simulink model "SafaeeModel"  (R2021a)
settings: Solver=VariableStepAuto  StartTime=0.0  StopTime=10  RelTol=1e-3
libraries: fuzblock x6
settings Model: Creator=carlos  LastModifiedBy=Lenovo
settings SolverCC: AlgebraicLoopSolver=TrustRegion
settings DataIOCC: ReturnWorkspaceOutputs=off
settings DebuggingCC: SFMachineParentedDataDiag=warning  ArithmeticOperatorsInVariantConditions=warning
settings SFSimCC: CustomCodeUndefinedFunction=UseInterfaceOnly

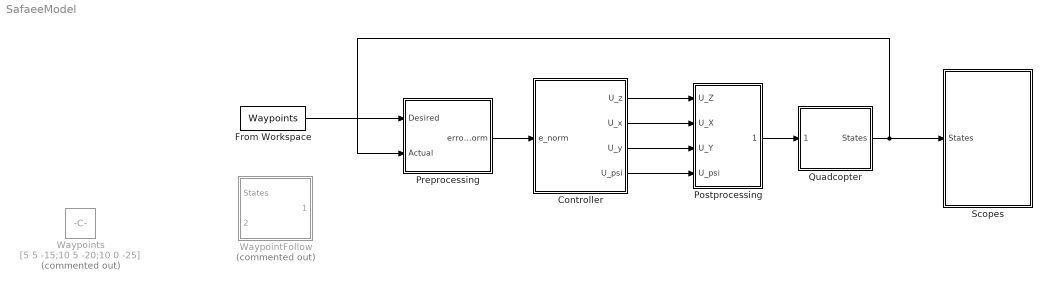
== system SafaeeModel ==
  Controller : Subsystem
  From Workspace : FromWorkspace  VariableName=Waypoints
  Postprocessing : Subsystem
  Preprocessing : Subsystem
  Quadcopter : Subsystem
  Scopes : Subsystem
  WaypointFollow : Subsystem  Commented=on
  Waypoints : Constant  Commented=on  Value=[5 5 -15;10 5 -20;10 0 -25]  VectorParams1D=off
  wires:
  Preprocessing/1(errorNorm) -> Controller/1(e_norm)
  Controller/1(U_z) -> Postprocessing/1(U_Z)
  Controller/2(U_x) -> Postprocessing/2(U_X)
  Controller/3(U_y) -> Postprocessing/3(U_Y)
  Controller/4(U_psi) -> Postprocessing/4(U_psi)
  Postprocessing/1(Omegas) -> Quadcopter/1(Omegas)
  Quadcopter/1(States) -> Preprocessing/2(Actual), Scopes/1(States)
  From Workspace/1 -> Preprocessing/1(Desired)

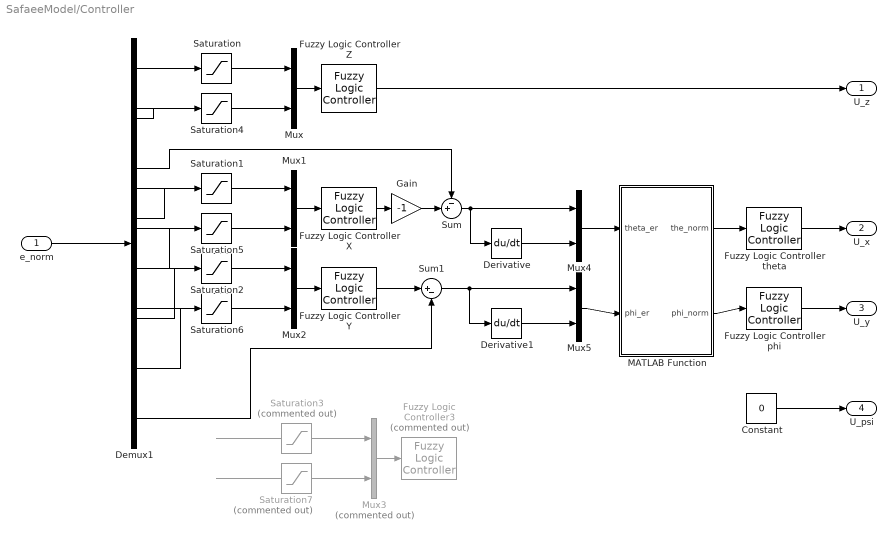
== system SafaeeModel/Controller ==
  e_norm : Inport
  Constant : Constant  Value=0
  Demux1 : Demux  Outputs=8
  Derivative : Derivative  CoefficientInTFapproximation=1
  Derivative1 : Derivative  CoefficientInTFapproximation=1
  Fuzzy Logic Controller X : fuzblock/Fuzzy Logic  Controller  FIS=FLCs.FLC_X  OutputSampleNumber=101  DataType=double  FuzzifiedInputs=off  RuleFiringStrengths=off  RuleOutputs=off  AggregatedOutputs=off  SimulateUsing=Interpreted execution  OutOfRangeInputValueMessage=warning  NoRuleFiredMessage=warning  EmptyOutputFuzzySetMessage=warning
  Fuzzy Logic Controller Y : fuzblock/Fuzzy Logic  Controller  FIS=FLCs.FLC_Y  OutputSampleNumber=101  DataType=double  FuzzifiedInputs=off  RuleFiringStrengths=off  RuleOutputs=off  AggregatedOutputs=off  SimulateUsing=Interpreted execution  OutOfRangeInputValueMessage=warning  NoRuleFiredMessage=warning  EmptyOutputFuzzySetMessage=warning
  Fuzzy Logic Controller Z : fuzblock/Fuzzy Logic  Controller  FIS=FLCs.FLC_Z  OutputSampleNumber=101  DataType=double  FuzzifiedInputs=off  RuleFiringStrengths=off  RuleOutputs=off  AggregatedOutputs=off  SimulateUsing=Interpreted execution  OutOfRangeInputValueMessage=warning  NoRuleFiredMessage=warning  EmptyOutputFuzzySetMessage=warning
  Fuzzy Logic Controller phi : fuzblock/Fuzzy Logic  Controller  FIS=FLCs.FLC_phi  OutputSampleNumber=101  DataType=double  FuzzifiedInputs=off  RuleFiringStrengths=off  RuleOutputs=off  AggregatedOutputs=off  SimulateUsing=Interpreted execution  OutOfRangeInputValueMessage=warning  NoRuleFiredMessage=warning  EmptyOutputFuzzySetMessage=warning
  Fuzzy Logic Controller theta : fuzblock/Fuzzy Logic  Controller  FIS=FLCs.FLC_th  OutputSampleNumber=101  DataType=double  FuzzifiedInputs=off  RuleFiringStrengths=off  RuleOutputs=off  AggregatedOutputs=off  SimulateUsing=Interpreted execution  OutOfRangeInputValueMessage=warning  NoRuleFiredMessage=warning  EmptyOutputFuzzySetMessage=warning
  Fuzzy Logic Controller3 : fuzblock/Fuzzy Logic  Controller  Commented=on  FIS=FLCs.FLC_psi  OutputSampleNumber=101  DataType=double  FuzzifiedInputs=off  RuleFiringStrengths=off  RuleOutputs=off  AggregatedOutputs=off  SimulateUsing=Interpreted execution  OutOfRangeInputValueMessage=warning  NoRuleFiredMessage=warning  EmptyOutputFuzzySetMessage=warning
  Gain : Gain  Gain=-1
  MATLAB Function : MATLAB Function  TreatAsAtomicUnit=on
  Mux{,1..2,4..5} (5 alike) : Mux  Inputs=2
  Mux3 : Mux  Commented=on  Inputs=2
  Saturation : Saturate  UpperLimit=1  LowerLimit=-1  ZeroCross=off
  Saturation1 : Saturate  UpperLimit=1  LowerLimit=-1  ZeroCross=off
  Saturation2 : Saturate  UpperLimit=1  LowerLimit=-1  ZeroCross=off
  Saturation3 : Saturate  Commented=on  UpperLimit=1  LowerLimit=-1  ZeroCross=off
  Saturation4 : Saturate  UpperLimit=3  LowerLimit=-3  ZeroCross=off
  Saturation5 : Saturate  UpperLimit=3  LowerLimit=-3  ZeroCross=off
  Saturation6 : Saturate  UpperLimit=3  LowerLimit=-3  ZeroCross=off
  Saturation7 : Saturate  Commented=on  UpperLimit=3  LowerLimit=-3  ZeroCross=off
  Sum : Sum  Inputs=-+|
  Sum1 : Sum  Inputs=|+-
  U_z : Outport  VectorParamsAs1DForOutWhenUnconnected=off
  U_x : Outport  Port=2  VectorParamsAs1DForOutWhenUnconnected=off
  U_y : Outport  Port=3  VectorParamsAs1DForOutWhenUnconnected=off
  U_psi : Outport  Port=4  VectorParamsAs1DForOutWhenUnconnected=off
  wires:
  Fuzzy Logic Controller Z/1 -> U_z/1
  Demux1/3 -> Sum/1
  Demux1/4 -> Saturation1/1
  Demux1/5 -> Saturation5/1
  Demux1/2 -> Saturation4/1
  e_norm/1 -> Demux1/1
  Demux1/1 -> Saturation/1
  Demux1/6 -> Saturation2/1
  Demux1/8 -> Sum1/2
  Demux1/7 -> Saturation6/1
  Fuzzy Logic Controller X/1 -> Gain/1
  Sum/1 -> Mux4/1, Derivative/1
  Fuzzy Logic Controller theta/1 -> U_x/1
  Fuzzy Logic Controller Y/1 -> Sum1/1
  Sum1/1 -> Mux5/1, Derivative1/1
  Fuzzy Logic Controller phi/1 -> U_y/1
  Mux/1 -> Fuzzy Logic Controller Z/1
  Mux2/1 -> Fuzzy Logic Controller Y/1
  Mux1/1 -> Fuzzy Logic Controller X/1
  Mux3/1 -> Fuzzy Logic Controller3/1
  Derivative/1 -> Mux4/2
  Mux4/1 -> MATLAB Function/1(theta_er)
  Derivative1/1 -> Mux5/2
  Mux5/1 -> MATLAB Function/2(phi_er)
  MATLAB Function/1(the_norm) -> Fuzzy Logic Controller theta/1
  MATLAB Function/2(phi_norm) -> Fuzzy Logic Controller phi/1
  Gain/1 -> Sum/2
  Saturation/1 -> Mux/1
  Saturation1/1 -> Mux1/1
  Saturation2/1 -> Mux2/1
  Saturation3/1 -> Mux3/1
  Saturation4/1 -> Mux/2
  Saturation5/1 -> Mux1/2
  Saturation6/1 -> Mux2/2
  Saturation7/1 -> Mux3/2
  Constant/1 -> U_psi/1

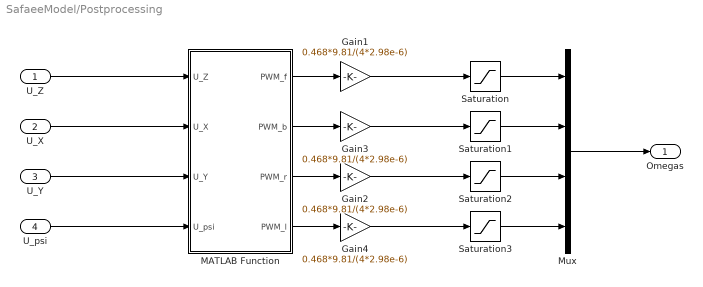
== system SafaeeModel/Postprocessing ==
  U_Z : Inport
  U_X : Inport  Port=2
  U_Y : Inport  Port=3
  U_psi : Inport  Port=4
  Gain{1..4} (4 alike) : Gain  Gain=0.468*9.81/(4*2.98e-6)
  MATLAB Function : MATLAB Function  TreatAsAtomicUnit=on
  Mux : Mux
  Saturation{,1..3} (4 alike) : Saturate  UpperLimit=1000000  LowerLimit=0  ZeroCross=off
  Omegas : Outport  VectorParamsAs1DForOutWhenUnconnected=off
  wires:
  Gain2/1 -> Saturation2/1
  Mux/1 -> Omegas/1
  Gain4/1 -> Saturation3/1
  MATLAB Function/4(PWM_l) -> Gain4/1
  MATLAB Function/2(PWM_b) -> Gain3/1
  Gain3/1 -> Saturation1/1
  MATLAB Function/3(PWM_r) -> Gain2/1
  Gain1/1 -> Saturation/1
  U_Y/1 -> MATLAB Function/3(U_Y)
  MATLAB Function/1(PWM_f) -> Gain1/1
  U_Z/1 -> MATLAB Function/1(U_Z)
  U_psi/1 -> MATLAB Function/4(U_psi)
  U_X/1 -> MATLAB Function/2(U_X)
  Saturation/1 -> Mux/1
  Saturation1/1 -> Mux/2
  Saturation2/1 -> Mux/3
  Saturation3/1 -> Mux/4

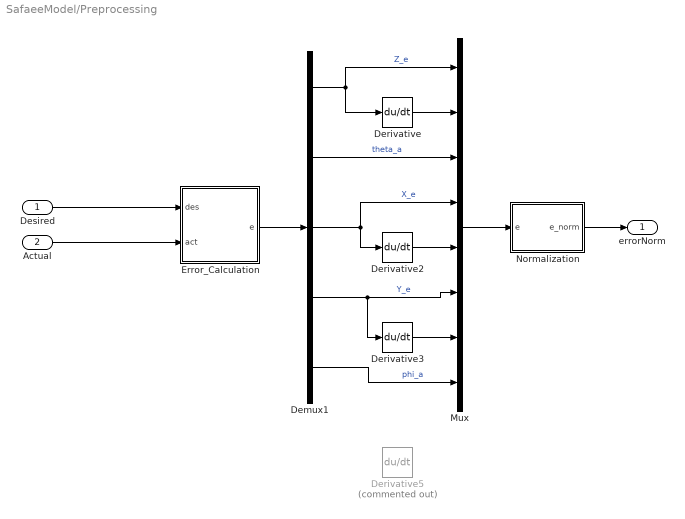
== system SafaeeModel/Preprocessing ==
  Desired : Inport
  Actual : Inport  Port=2
  Demux1 : Demux  Outputs=5
  Derivative : Derivative  CoefficientInTFapproximation=1
  Derivative2 : Derivative  CoefficientInTFapproximation=1
  Derivative3 : Derivative  CoefficientInTFapproximation=1
  Derivative5 : Derivative  Commented=on  CoefficientInTFapproximation=1
  Error_Calculation : MATLAB Function  TreatAsAtomicUnit=on
  Mux : Mux  Inputs=8
  Normalization : MATLAB Function  TreatAsAtomicUnit=on
  errorNorm : Outport  VectorParamsAs1DForOutWhenUnconnected=off
  wires:
  Demux1/1 -> Mux/1, Derivative/1  "Z_e"
  Demux1/2 -> Mux/3  "theta_a"
  Demux1/3 -> Mux/4, Derivative2/1  "X_e"
  Error_Calculation/1(e) -> Demux1/1
  Normalization/1(e_norm) -> errorNorm/1
  Demux1/4 -> Derivative3/1, Mux/6  "Y_e"
  Demux1/5 -> Mux/8  "phi_a"
  Mux/1 -> Normalization/1(e)
  Derivative2/1 -> Mux/5
  Derivative3/1 -> Mux/7
  Derivative/1 -> Mux/2
  Desired/1 -> Error_Calculation/1(des)
  Actual/1 -> Error_Calculation/2(act)

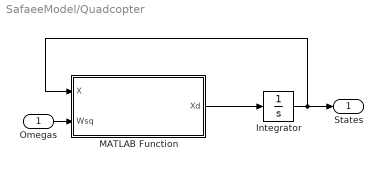
== system SafaeeModel/Quadcopter ==
  Omegas : Inport
  Integrator : Integrator  InitialCondition=[0;0;0;0;0;0;0;0;0;0;0;0]
  MATLAB Function : MATLAB Function  TreatAsAtomicUnit=on
  States : Outport  VectorParamsAs1DForOutWhenUnconnected=off
  wires:
  Omegas/1 -> MATLAB Function/2(Wsq)
  MATLAB Function/1(Xd) -> Integrator/1
  Integrator/1 -> States/1, MATLAB Function/1(X)

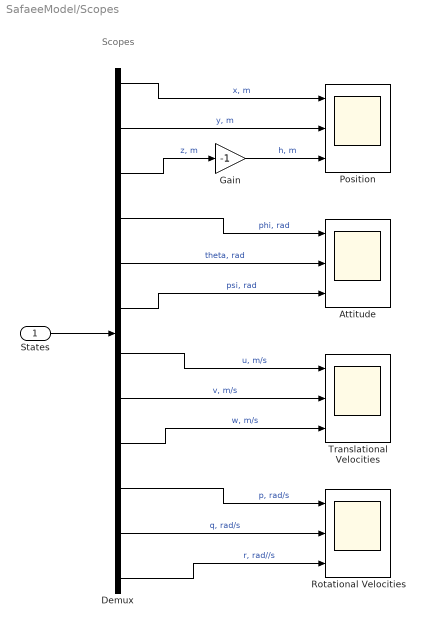
== system SafaeeModel/Scopes ==
  note: Scopes
  States : Inport
  Attitude : Scope  NumInputPorts=3
  Demux : Demux  Outputs=12
  Gain : Gain  Gain=-1
  Position : Scope  NumInputPorts=3
  Rotational Velocities : Scope  NumInputPorts=3
  Translational Velocities : Scope  NumInputPorts=3
  wires:
  Demux/5 -> Attitude/2  "theta, rad"
  Demux/1 -> Position/1  "x, m"
  Demux/4 -> Attitude/1  "phi, rad"
  Gain/1 -> Position/3  "h, m"
  Demux/6 -> Attitude/3  "psi, rad"
  Demux/11 -> Rotational Velocities/2  "q, rad/s"
  States/1 -> Demux/1
  Demux/3 -> Gain/1  "z, m"
  Demux/10 -> Rotational Velocities/1  "p, rad/s"
  Demux/12 -> Rotational Velocities/3  "r, rad//s"
  Demux/9 -> Translational Velocities/3  "w, m/s"
  Demux/8 -> Translational Velocities/2  "v, m/s"
  Demux/7 -> Translational Velocities/1  "u, m/s"
  Demux/2 -> Position/2  "y, m"

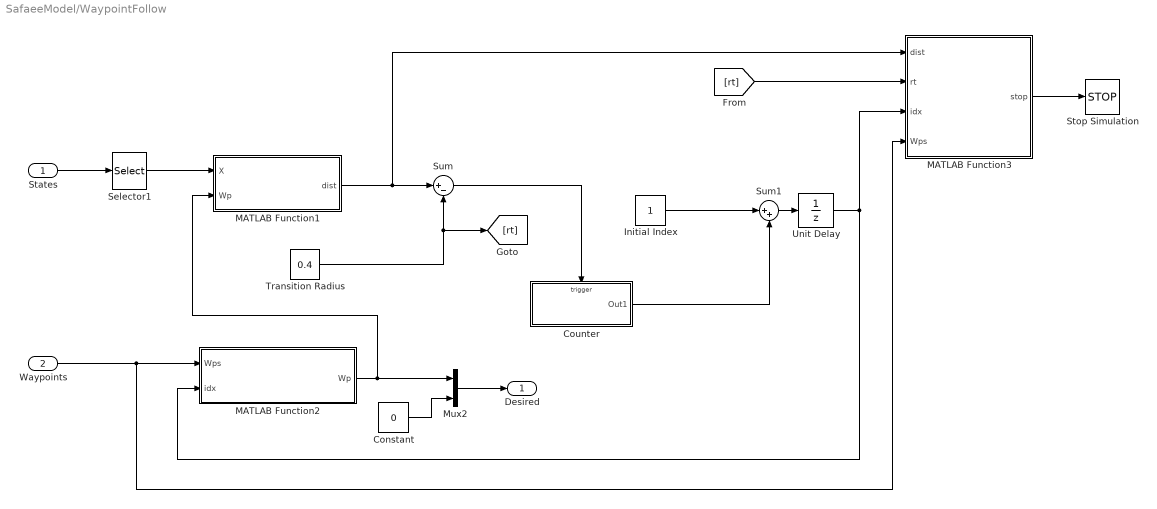
== system SafaeeModel/WaypointFollow ==
  States : Inport
  Waypoints : Inport  Port=2
  Constant : Constant  Value=0
  Counter : Subsystem  TreatAsAtomicUnit=on
  Initial Index : Constant
  MATLAB Function1 : MATLAB Function  TreatAsAtomicUnit=on
  MATLAB Function2 : MATLAB Function  TreatAsAtomicUnit=on
  MATLAB Function3 : MATLAB Function  TreatAsAtomicUnit=on
  Mux2 : Mux  Inputs=2
  Selector1 : Selector  InputPortWidth=12  IndexOptions=Index vector (dialog)  Indices=[1 2 3]  OutputSizes=1
  Stop Simulation : Stop
  Sum : Sum  Inputs=|+-
  Sum1 : Sum  Inputs=|++
  Transition Radius : Constant  Value=0.4
  Unit Delay : UnitDelay  InitialCondition=1  SampleTime=-1  HasFrameUpgradeWarning=on
  Desired : Outport
  wires:
  States/1 -> Selector1/1
  Selector1/1 -> MATLAB Function1/1(X)
  Transition Radius/1 -> [rt], Sum/2
  Sum/1 -> Counter/Trigger
  Counter/1(Out1) -> Sum1/2
  Initial Index/1 -> Sum1/1
  MATLAB Function2/1(Wp) -> Mux2/1, MATLAB Function1/2(Wp)
  Sum1/1 -> Unit Delay/1
  [rt] -> MATLAB Function3/2(rt)
  Waypoints/1 -> MATLAB Function2/1(Wps), MATLAB Function3/4(Wps)
  MATLAB Function3/1(stop) -> Stop Simulation/1
  Mux2/1 -> Desired/1
  Constant/1 -> Mux2/2
  Unit Delay/1 -> MATLAB Function2/2(idx), MATLAB Function3/3(idx)
  MATLAB Function1/1(dist) -> MATLAB Function3/1(dist), Sum/1

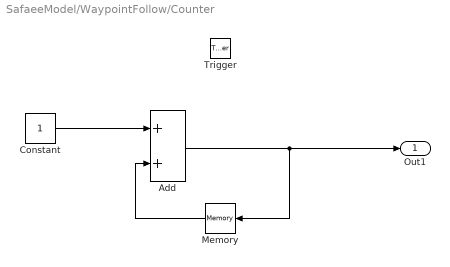
== system SafaeeModel/WaypointFollow/Counter ==
  Trigger : TriggerPort  TriggerType=falling  VariantControl=(inherit)
  Add : Sum
  Constant : Constant
  Memory : Memory  InheritSampleTime=on
  Out1 : Outport
  wires:
  Constant/1 -> Add/1
  Add/1 -> Memory/1, Out1/1
  Memory/1 -> Add/2

== matlab function SafaeeModel/Preprocessing/Error_Calculation ==
  data: des input; e output; act input
function e = fcn(des, act)

X_des = des(1,1); Y_des = des(1,2); Z_des = des(1,3);
% phi_des = des(4,1); theta_des = des(5,1); 
% psi_des = des(4,1);

X_act = act(1,1); Y_act = act(2,1); Z_act = act(3,1);
phi_act = act(4,1); theta_act = act(5,1); 
% psi_act = act(6,1);

ex      = X_des - X_act;
ey      = Y_des - Y_act;
ez      = Z_des - Z_act;
% ephi    = phi_des - phi_act;
% etheta  = theta_des - theta_act;
% epsi    = psi_des - psi_act;

e = [ez; theta_act; ex; ey; phi_act];% epsi];

== matlab function SafaeeModel/Quadcopter/MATLAB Function ==
  data: X input; Xd output; Wsq input
function Xd = Quadcopter(X, Wsq)
% Parameters from Luukkonen
g = 9.81;
M = 0.468;
Jx = 4.856e-3;
Jy = 4.856e-3;
Jz = 8.801e-3;
l = 0.225;
KT = 2.980e-6;
Kt = 1.140e-7;

% States
x   = X(1,1);  y   = X(2,1);  z   = X(3,1);
phi = X(4,1);  the = X(5,1);  psi = X(6,1);
u   = X(7,1);  v   = X(8,1);  w   = X(9,1);
p   = X(10,1); q   = X(11,1); r   = X(12,1);

% Motor Forces (front, back, right, left)
Tf   = KT*Wsq(1,1);  Tb   = KT*Wsq(2,1);   Tr   = KT*Wsq(3,1);  Tl   = KT*Wsq(4,1);

% Motor Torques (front, back, right, left)
tauf = -Kt*Wsq(1,1);  taub = -Kt*Wsq(2,1);  taur = Kt*Wsq(3,1);  taul = Kt*Wsq(4,1);

%% Safaee's quadcopter model
% Elements of Rotation Matrix from Inertial frame to Body Frame (Transposed)
R11 = cos(phi)*cos(psi);
R12 = sin(phi)*sin(the)*cos(psi) - cos(phi)*sin(psi);
R13 = cos(phi)*sin(the)*cos(psi) + sin(phi)*sin(psi);
R21 = cos(the)*sin(psi);
R22 = sin(phi)*sin(the)*sin(psi) + cos(phi)*cos(psi);
R23 = cos(phi)*sin(the)*sin(psi) - sin(phi)*cos(psi);
R31 = -sin(the);
R32 = sin(phi)*cos(the);
R33 = cos(phi)*cos(the);

% Rotation Matrix from Inertial frame to Body Frame (Transposed)
RI2BT = [R11 R12 R13;
         R21 R22 R23;
         R31 R32 R33];

% Translational Kinematics
Xd1 = RI2BT*[u; v; w];

% Elements of Rotational Kinematics Matrix
RE1 = 1;
RE2 = sin(phi)*tan(the);
RE3 = cos(phi)*tan(the);
RE4 = 0;
RE5 = cos(phi);
RE6 = -sin(phi);
RE7 = 0;
RE8 = sin(phi)./cos(the);
RE9 = cos(phi)./cos(the);

% Rotational Kinematics Matrix
RE = [RE1 RE2 RE3;
      RE4 RE5 RE6;
      RE7 RE8 RE9];
  
% Rotational Kinematics
Xd2 = RE*[p; q; r];

% Total Thrust
Tt = Tf + Tb + Tr + Tl;

% Total Torque along x axis
Tphi = l*(Tl - Tr);

% Total Torque along y axis
Tthe = l*(Tf - Tb);

% Total Torque along z axis
Tpsi = tauf + taub + taur + taul;

% Translational Dynamics
ud = r*v - q*w - g*sin(the);
vd = p*w - r*u + g*sin(phi)*cos(the);
wd = q*u - p*v + g*cos(phi)*cos(the) - Tt/M;

if abs(ud) < 1e-10
    ud = 0;
end

if abs(vd) < 1e-10
    vd = 0;
end

if abs(wd) < 1e-10
    wd = 0;
end

Xd3 = [ud; vd; wd];

% Rotational Dynamics
pd = q*r*(Jy - Jz)/Jx + Tphi/Jx;
qd = p*r*(Jz - Jx)/Jy + Tthe/Jy;
rd = p*q*(Jx - Jy)/Jz + Tpsi/Jz;

if abs(pd) < 1e-10
    pd = 0;
end

if abs(qd) < 1e-10
    qd = 0;
end

if abs(rd) < 1e-10
    rd = 0;
end

Xd4 = [pd; qd; rd];

Xd = [Xd1; Xd2; Xd3; Xd4];

== matlab function SafaeeModel/Preprocessing/Normalization ==
  data: e input; e_norm output
function e_norm = Normalization(e)

Z_e = e(1,1); 
Z_ed = e(2,1); 

theta_a = e(3,1);

X_e = e(4,1); 
X_ed = e(5,1);

Y_e = e(6,1);
Y_ed = e(7,1);

phi_a = e(8,1);

% psi_e = e(9,1);
% psi_ed = e(10,1);

X_max = 10; Y_max = 10; Z_max = 50;
Xd_max = 30; Yd_max = 30; Zd_max = 30;
% psi_max = pi/3;
% psid_max = pi/6;

Xe_norm = X_e/X_max;
Ye_norm = Y_e/Y_max;
Ze_norm = Z_e/Z_max;
% phie_norm = phi_a/phi_max;
% thetae_norm = theta_a/theta_max;
% psie_norm = psi_e/psi_max;

Xed_norm = 3*X_ed/Xd_max;
Yed_norm = 3*Y_ed/Yd_max;
Zed_norm = 3*Z_ed/Zd_max;
% psied_norm = 3*psi_ed/psid_max;

e_norm = [Ze_norm; Zed_norm; theta_a; Xe_norm; Xed_norm; Ye_norm; Yed_norm;
    phi_a];% psie_norm; psied_norm];

== matlab function SafaeeModel/Postprocessing/MATLAB Function ==
  data: U_Z input; PWM_f output; PWM_b output; U_X input; U_Y input; U_psi input; PWM_r output; PWM_l output
function [PWM_f, PWM_b, PWM_r, PWM_l] = fcn(U_Z, U_X, U_Y, U_psi)

PWM_f = 2*(-U_Z + U_X - U_psi) + 1;
PWM_r = 2*(-U_Z - U_Y + U_psi) + 1;
PWM_b = 2*(-U_Z - U_X - U_psi) + 1;
PWM_l = 2*(-U_Z + U_Y + U_psi) + 1;

== matlab function SafaeeModel/Controller/MATLAB Function ==
  data: theta_er input; the_norm output; phi_er input; phi_norm output
function [the_norm, phi_norm] = fcn(theta_er, phi_er)

theta_e = theta_er(1,1);
theta_ed = theta_er(2,1);

phi_e = phi_er(1,1);
phi_ed = phi_er(2,1);

phi_max = pi/3; theta_max  = pi/3;
phid_max = pi/6; thetad_max  = pi/6;

phie_norm = min(max(phi_e/phi_max, -1), 1);
thetae_norm = min(max(theta_e/theta_max, -1), 1);

phied_norm = min(max(3*phi_ed/phid_max, -3), 3);
thetaed_norm = min(max(3*theta_ed/thetad_max, -3), 3);

the_norm = [thetae_norm; thetaed_norm];
phi_norm = [phie_norm; phied_norm];

== matlab function SafaeeModel/WaypointFollow/MATLAB Function1 ==
  data: X input; dist output; Wp input
function dist = distance(X, Wp)

dist = sqrt((Wp(1) - X(1))^2 + (Wp(2) - X(2))^2 + (Wp(3) - X(3))^2);

== matlab function SafaeeModel/WaypointFollow/MATLAB Function2 ==
  data: Wps input; Wp output; idx input
function Wp = ChooseWaypoint(Wps, idx)

Wp = Wps(idx,:)';

== matlab function SafaeeModel/WaypointFollow/MATLAB Function3 ==
  data: dist input; stop output; rt input; idx input; Wps input
function stop = StopAtLastWp(dist, rt, idx, Wps)

[m,~] = size(Wps);

if idx == m && (dist - rt) <= 5e-2
    stop = 1;
else
    stop = 0;
end
